simulink model "second"  (R2020a)
settings: Solver=VariableStepAuto  StartTime=0.0  StopTime=100  RelTol=1e-3
model workspace (MAT data in the model file):
  K1 = Simulink.Parameter
  K1.Value = 50
  K1.DataType = 'auto'
  K1.Dimensions = [1 1]
  K2 = Simulink.Parameter
  K2.Value = 2000
  K2.DataType = 'auto'
  K2.Dimensions = [1 1]
  M1 = Simulink.Parameter
  M1.Value = 100
  M1.DataType = 'auto'
  M1.Dimensions = [1 1]
  M2 = Simulink.Parameter
  M2.Value = 50
  M2.DataType = 'auto'
  M2.Dimensions = [1 1]
  b = Simulink.Parameter
  b.Value = 50
  b.DataType = 'auto'
  b.Dimensions = [1 1]
settings Model: Creator=Admin  LastModifiedBy=Admin

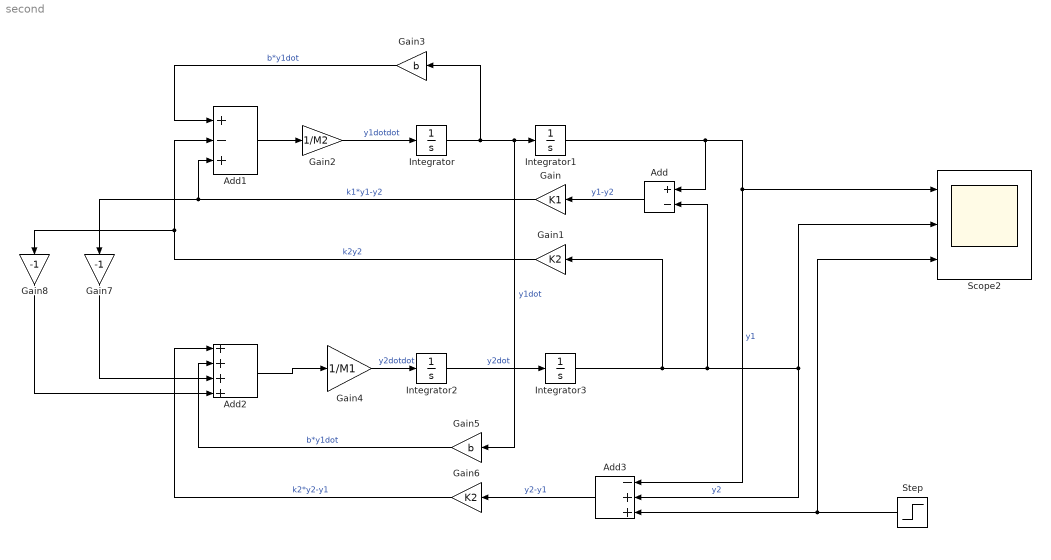
== system second ==
  Add : Sum  Inputs=+-
  Add1 : Sum  Inputs=+-+
  Add2 : Sum  Inputs=++++
  Add3 : Sum  Inputs=-++
  Gain : Gain  Gain=K1
  Gain1 : Gain  Gain=K2
  Gain2 : Gain  Gain=1/M2
  Gain3 : Gain  Gain=b
  Gain4 : Gain  Gain=1/M1
  Gain5 : Gain  Gain=b
  Gain6 : Gain  Gain=K2
  Gain7 : Gain  Gain=-1
  Gain8 : Gain  Gain=-1
  Integrator{,1..3} (4 alike) : Integrator
  Scope2 : Scope  NumInputPorts=3
  Step : Step  SampleTime=0
  wires:
  Integrator1/1 -> Add/1, Add3/1, Scope2/1  "y1"
  Integrator/1 -> Gain3/1, Integrator1/1, Gain5/1  "y1dot"
  Gain2/1 -> Integrator/1  "y1dotdot"
  Integrator2/1 -> Integrator3/1  "y2dot"
  Integrator3/1 -> Gain1/1, Add/2, Add3/2, Scope2/2  "y2"
  Add/1 -> Gain/1  "y1-y2"
  Add1/1 -> Gain2/1
  Gain/1 -> Gain7/1, Add1/3  "k1*y1-y2"
  Gain1/1 -> Gain8/1, Add1/2  "k2y2"
  Gain3/1 -> Add1/1  "b*y1dot"
  Gain4/1 -> Integrator2/1  "y2dotdot"
  Add2/1 -> Gain4/1
  Gain5/1 -> Add2/2  "b*y1dot"
  Add3/1 -> Gain6/1  "y2-y1"
  Gain6/1 -> Add2/1  "k2*y2-y1"
  Step/1 -> Scope2/3, Add3/3
  Gain7/1 -> Add2/3
  Gain8/1 -> Add2/4
